simulink model "DRSsimulink"  (R2026a)
settings: Solver=FixedStepAuto  StopTime=141.85  FixedStep=0.05
InitFcn:
  | DRS
values from neighbouring files (symbols this model uses):
  AOAConv = AOAConversion(19:71,1)    [DRS.m]
  ServoConv = AOAConversion(19:71,2)    [DRS.m]
settings Model: Creator=Xxzer  LastModifiedBy=Xxzer
settings RTWCC: SystemTargetFile=ert.tlc  Description=Embedded Coder
settings ERTTargetCC: GenerateSampleERTMain=on

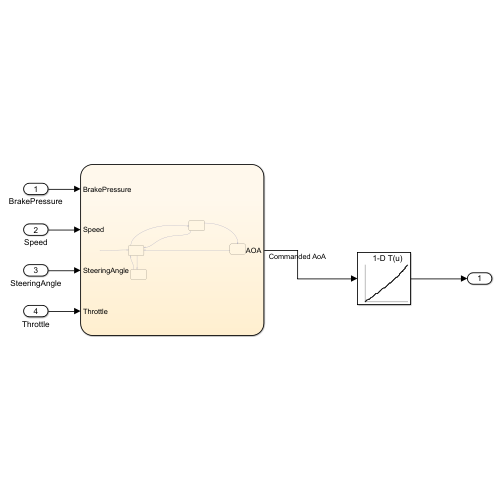
[thumbnail: Simulink's stored preview of the top-level diagram]
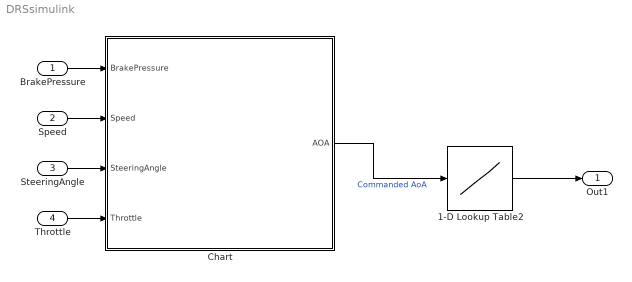
== system DRSsimulink ==
  BrakePressure : Inport
  Speed : Inport  Port=2
  SteeringAngle : Inport  Port=3
  Throttle : Inport  Port=4
  1-D Lookup Table2 : Lookup_n-D  NumberOfTableDimensions=1  BreakpointsForDimension1=ServoConv  Table=AOAConv  InternalRulePriority=Speed  RndMeth=Simplest
  Chart : Stateflow chart  TreatAsAtomicUnit=on
  Out1 : Outport
  wires:
  Chart/1(AOA) -> 1-D Lookup Table2/1  "Commanded AoA"
  1-D Lookup Table2/1 -> Out1/1
  BrakePressure/1 -> Chart/1(BrakePressure)
  Speed/1 -> Chart/2(Speed)
  Throttle/1 -> Chart/4(Throttle)
  SteeringAngle/1 -> Chart/3(SteeringAngle)

== stateflow chart DRSsimulink/Chart ==
  state DRSArming
  state DRS
    entry:
    AOA = 0.25;
  state Downforce
    entry:
    AOA = 14;
  state Aerobrake
    entry:
    AOA = 17.5;
  DRSArming -> DRS [order 1] : after(0.5,sec)
  Downforce -> DRSArming [order 1] : [Speed > 15 && Throttle > 95 && SteeringAngle < 5 && BrakePressure < 5]
  DRSArming -> Downforce [order 2] : [Throttle < 90 || SteeringAngle >= 10 || BrakePressure >= 5]
  (default) -> Downforce
  DRS -> Downforce : [Throttle < 90 || SteeringAngle >= 10 || BrakePressure >= 5]
  Aerobrake -> Downforce : [BrakePressure <= 15]
  Downforce -> Aerobrake [order 2] : [BrakePressure > 50]
  data: BrakePressure input; Speed input; SteeringAngle input; Throttle input; AOA output
